simulink model "quadcoptermodel_liniarize"  (R2017b)
settings: Solver=FixedStepAuto  StartTime=0.0  StopTime=10.0  FixedStep=0.0025  RelTol=1e-3

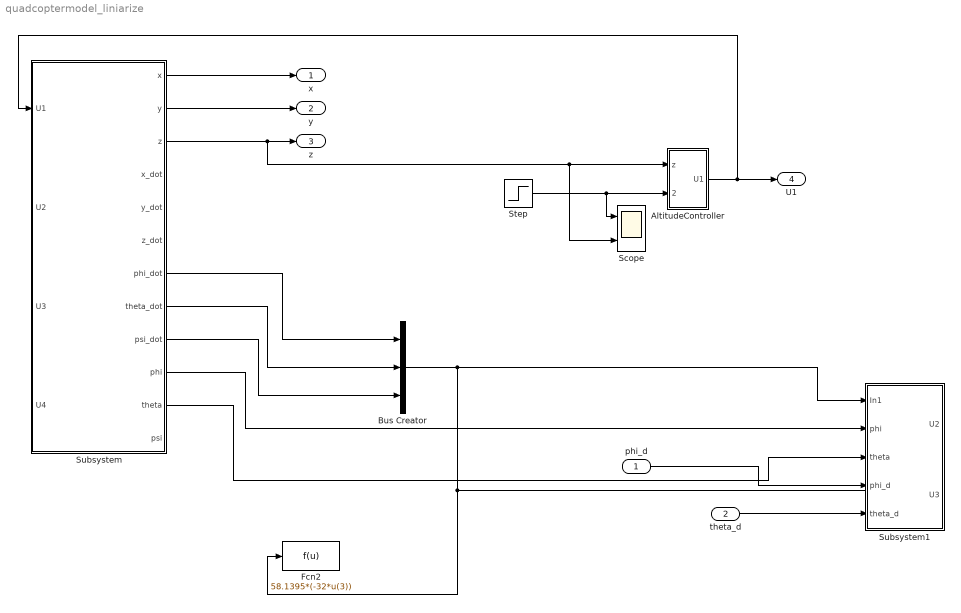
== system quadcoptermodel_liniarize ==
  phi_d : Inport
  theta_d : Inport  Port=2
  AltitudeController : Subsystem
  Bus Creator : BusCreator  Inputs=3
  Fcn2 : Fcn  Expr=58.1395*(-32*u(3))
  Scope : Scope  NumInputPorts=2
  Step : Step  SampleTime=0
  Subsystem : Subsystem
  Subsystem1 : Subsystem
  x : Outport
  y : Outport  Port=2
  z : Outport  Port=3
  U1 : Outport  Port=4
  wires:
  Subsystem/1(x) -> x/1
  Subsystem/2(y) -> y/1
  Subsystem/3(z) -> Scope/2, AltitudeController/1(z), z/1
  AltitudeController/1(U1) -> Subsystem/1(U1), U1/1
  Step/1 -> Scope/1, AltitudeController/2(z_d)
  Subsystem/7(phi_dot) -> Bus Creator/1
  Subsystem/8(theta_dot) -> Bus Creator/2
  Subsystem/9(psi_dot) -> Bus Creator/3
  Bus Creator/1 -> Subsystem1/1(In1), Fcn2/1
  Subsystem/10(phi) -> Subsystem1/2(phi)
  Subsystem/11(theta) -> Subsystem1/3(theta)
  phi_d/1 -> Subsystem1/4(phi_d)
  theta_d/1 -> Subsystem1/5(theta_d)

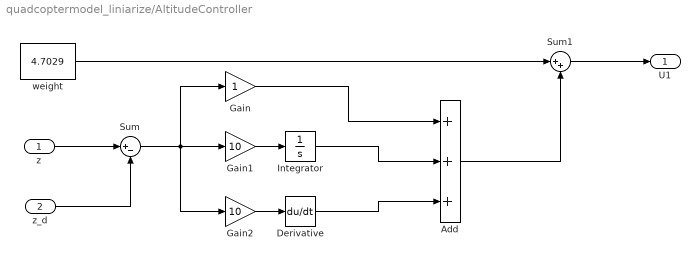
== system quadcoptermodel_liniarize/AltitudeController ==
  z : Inport
  z_d : Inport  Port=2
  Add : Sum  Inputs=+++
  Derivative : Derivative
  Gain : Gain
  Gain1 : Gain  Gain=10
  Gain2 : Gain  Gain=10
  Integrator : Integrator
  Sum : Sum  Inputs=|+-
  Sum1 : Sum  Inputs=|++
  weight : Constant  Value=4.7029
  U1 : Outport
  wires:
  Gain1/1 -> Integrator/1
  Sum/1 -> Gain/1, Gain1/1, Gain2/1
  weight/1 -> Sum1/1
  z_d/1 -> Sum/2
  Integrator/1 -> Add/2
  Add/1 -> Sum1/2
  Gain/1 -> Add/1
  Gain2/1 -> Derivative/1
  z/1 -> Sum/1
  Sum1/1 -> U1/1
  Derivative/1 -> Add/3

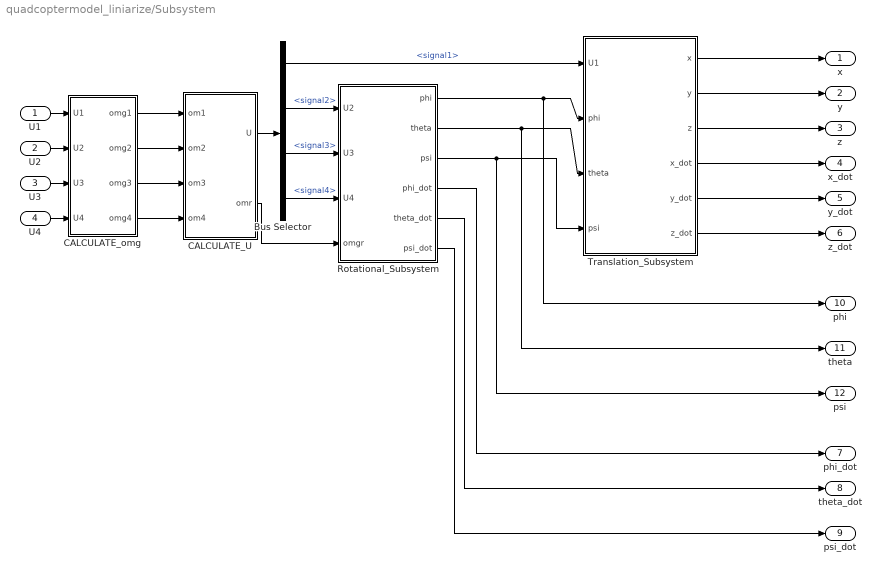
== system quadcoptermodel_liniarize/Subsystem ==
  U1 : Inport
  U2 : Inport  Port=2
  U3 : Inport  Port=3
  U4 : Inport  Port=4
  Bus Selector : BusSelector  OutputSignals=signal1,signal2,signal3,signal4
  CALCULATE_U : Subsystem
  CALCULATE_omg : Subsystem
  Rotational_Subsystem : Subsystem
  Translation_Subsystem : Subsystem
  x : Outport
  y : Outport  Port=2
  z : Outport  Port=3
  x_dot : Outport  Port=4
  y_dot : Outport  Port=5
  z_dot : Outport  Port=6
  phi_dot : Outport  Port=7
  theta_dot : Outport  Port=8
  psi_dot : Outport  Port=9
  phi : Outport  Port=10
  theta : Outport  Port=11
  psi : Outport  Port=12
  wires:
  CALCULATE_omg/1(omg1) -> CALCULATE_U/1(om1)
  CALCULATE_omg/4(omg4) -> CALCULATE_U/4(om4)
  CALCULATE_omg/2(omg2) -> CALCULATE_U/2(om2)
  CALCULATE_U/1(U) -> Bus Selector/1
  CALCULATE_omg/3(omg3) -> CALCULATE_U/3(om3)
  Rotational_Subsystem/1(phi) -> phi/1, Translation_Subsystem/2(phi)
  Rotational_Subsystem/2(theta) -> theta/1, Translation_Subsystem/3(theta)
  Rotational_Subsystem/3(psi) -> psi/1, Translation_Subsystem/4(psi)
  Translation_Subsystem/1(x) -> x/1
  Bus Selector/1 -> Translation_Subsystem/1(U1)  "<signal1>"
  Translation_Subsystem/2(y) -> y/1
  Translation_Subsystem/3(z) -> z/1
  Bus Selector/3 -> Rotational_Subsystem/2(U3)  "<signal3>"
  Bus Selector/4 -> Rotational_Subsystem/3(U4)  "<signal4>"
  CALCULATE_U/2(omr) -> Rotational_Subsystem/4(omgr)
  Bus Selector/2 -> Rotational_Subsystem/1(U2)  "<signal2>"
  Translation_Subsystem/6(z_dot) -> z_dot/1
  Translation_Subsystem/4(x_dot) -> x_dot/1
  U3/1 -> CALCULATE_omg/3(U3)
  Rotational_Subsystem/5(theta_dot) -> theta_dot/1
  U4/1 -> CALCULATE_omg/4(U4)
  U2/1 -> CALCULATE_omg/2(U2)
  U1/1 -> CALCULATE_omg/1(U1)
  Translation_Subsystem/5(y_dot) -> y_dot/1
  Rotational_Subsystem/6(psi_dot) -> psi_dot/1
  Rotational_Subsystem/4(phi_dot) -> phi_dot/1

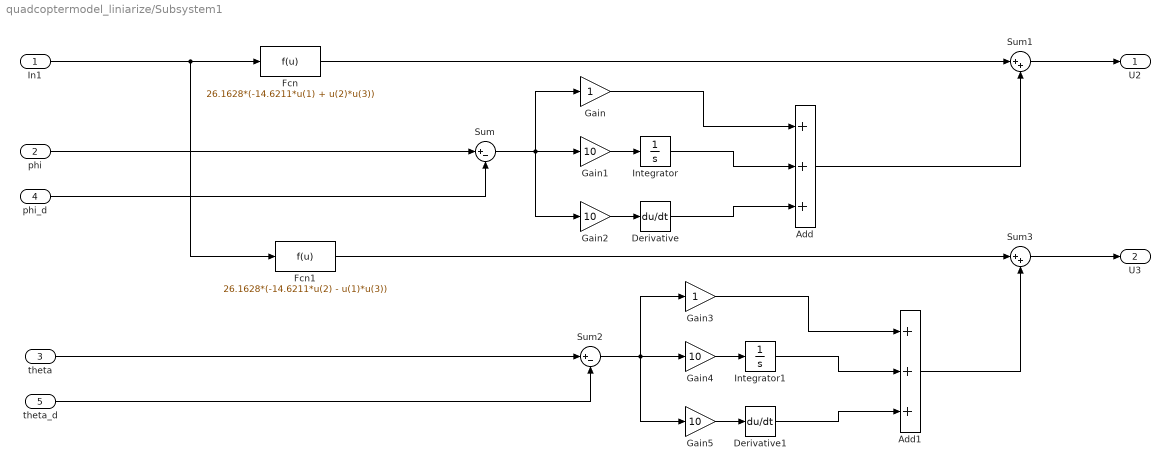
== system quadcoptermodel_liniarize/Subsystem1 ==
  In1 : Inport
  phi : Inport  Port=2
  theta : Inport  Port=3
  phi_d : Inport  Port=4
  theta_d : Inport  Port=5
  Add : Sum  Inputs=+++
  Add1 : Sum  Inputs=+++
  Derivative : Derivative
  Derivative1 : Derivative
  Fcn : Fcn  Expr=26.1628*(-14.6211*u(1) + u(2)*u(3))
  Fcn1 : Fcn  Expr=26.1628*(-14.6211*u(2) - u(1)*u(3))
  Gain : Gain
  Gain{1..2,4..5} (4 alike) : Gain  Gain=10
  Gain3 : Gain
  Integrator : Integrator
  Integrator1 : Integrator
  Sum : Sum  Inputs=|+-
  Sum1 : Sum  Inputs=|++
  Sum2 : Sum  Inputs=|+-
  Sum3 : Sum  Inputs=|++
  U2 : Outport
  U3 : Outport  Port=2
  wires:
  In1/1 -> Fcn1/1, Fcn/1
  theta_d/1 -> Sum2/2
  Integrator1/1 -> Add1/2
  Fcn1/1 -> Sum3/1
  Derivative1/1 -> Add1/3
  theta/1 -> Sum2/1
  Gain4/1 -> Integrator1/1
  Add1/1 -> Sum3/2
  Gain5/1 -> Derivative1/1
  Sum2/1 -> Gain3/1, Gain4/1, Gain5/1
  Sum3/1 -> U3/1
  Gain3/1 -> Add1/1
  Add/1 -> Sum1/2
  Integrator/1 -> Add/2
  phi_d/1 -> Sum/2
  Derivative/1 -> Add/3
  Gain/1 -> Add/1
  Gain2/1 -> Derivative/1
  Gain1/1 -> Integrator/1
  Sum/1 -> Gain/1, Gain1/1, Gain2/1
  Sum1/1 -> U2/1
  phi/1 -> Sum/1
  Fcn/1 -> Sum1/1

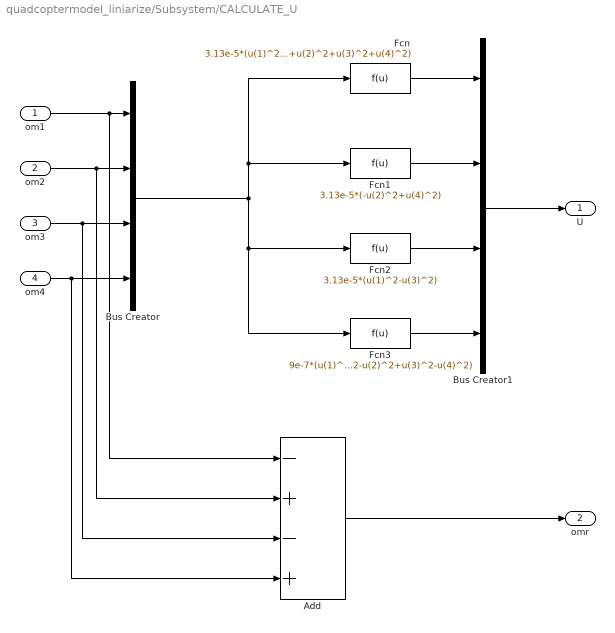
== system quadcoptermodel_liniarize/Subsystem/CALCULATE_U ==
  om1 : Inport
  om2 : Inport  Port=2
  om3 : Inport  Port=3
  om4 : Inport  Port=4
  Add : Sum  Inputs=-+-+
  Bus Creator : BusCreator  Inputs=4
  Bus Creator1 : BusCreator  Inputs=4
  Fcn : Fcn  Expr=3.13e-5*(u(1)^2+u(2)^2+u(3)^2+u(4)^2)
  Fcn1 : Fcn  Expr=3.13e-5*(-u(2)^2+u(4)^2)
  Fcn2 : Fcn  Expr=3.13e-5*(u(1)^2-u(3)^2)
  Fcn3 : Fcn  Expr=9e-7*(u(1)^2-u(2)^2+u(3)^2-u(4)^2)
  U : Outport
  omr : Outport  Port=2
  wires:
  Bus Creator1/1 -> U/1
  om3/1 -> Add/3, Bus Creator/3
  om1/1 -> Add/1, Bus Creator/1
  Bus Creator/1 -> Fcn3/1, Fcn2/1, Fcn1/1, Fcn/1
  Fcn1/1 -> Bus Creator1/2
  om4/1 -> Add/4, Bus Creator/4
  Fcn/1 -> Bus Creator1/1
  Fcn2/1 -> Bus Creator1/3
  om2/1 -> Add/2, Bus Creator/2
  Fcn3/1 -> Bus Creator1/4
  Add/1 -> omr/1

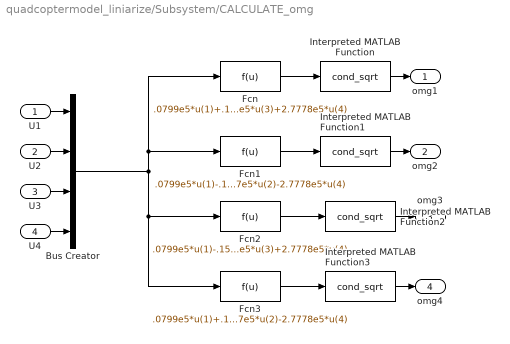
== system quadcoptermodel_liniarize/Subsystem/CALCULATE_omg ==
  U1 : Inport
  U2 : Inport  Port=2
  U3 : Inport  Port=3
  U4 : Inport  Port=4
  Bus Creator : BusCreator  Inputs=4
  Fcn : Fcn  Expr=.0799e5*u(1)+.1597e5*u(3)+2.7778e5*u(4)
  Fcn1 : Fcn  Expr=.0799e5*u(1)-.1597e5*u(2)-2.7778e5*u(4)
  Fcn2 : Fcn  Expr=.0799e5*u(1)-.1597e5*u(3)+2.7778e5*u(4)
  Fcn3 : Fcn  Expr=.0799e5*u(1)+.1597e5*u(2)-2.7778e5*u(4)
  Interpreted MATLAB Function{,1..3} (4 alike) : MATLABFcn  MATLABFcn=cond_sqrt
  omg1 : Outport
  omg2 : Outport  Port=2
  omg3 : Outport  Port=3
  omg4 : Outport  Port=4
  wires:
  Fcn/1 -> Interpreted MATLAB Function/1
  Fcn3/1 -> Interpreted MATLAB Function3/1
  U3/1 -> Bus Creator/3
  U4/1 -> Bus Creator/4
  Interpreted MATLAB Function/1 -> omg1/1
  Interpreted MATLAB Function3/1 -> omg4/1
  Interpreted MATLAB Function2/1 -> omg3/1
  Interpreted MATLAB Function1/1 -> omg2/1
  U1/1 -> Bus Creator/1
  U2/1 -> Bus Creator/2
  Fcn1/1 -> Interpreted MATLAB Function1/1
  Fcn2/1 -> Interpreted MATLAB Function2/1
  Bus Creator/1 -> Fcn2/1, Fcn3/1, Fcn1/1, Fcn/1

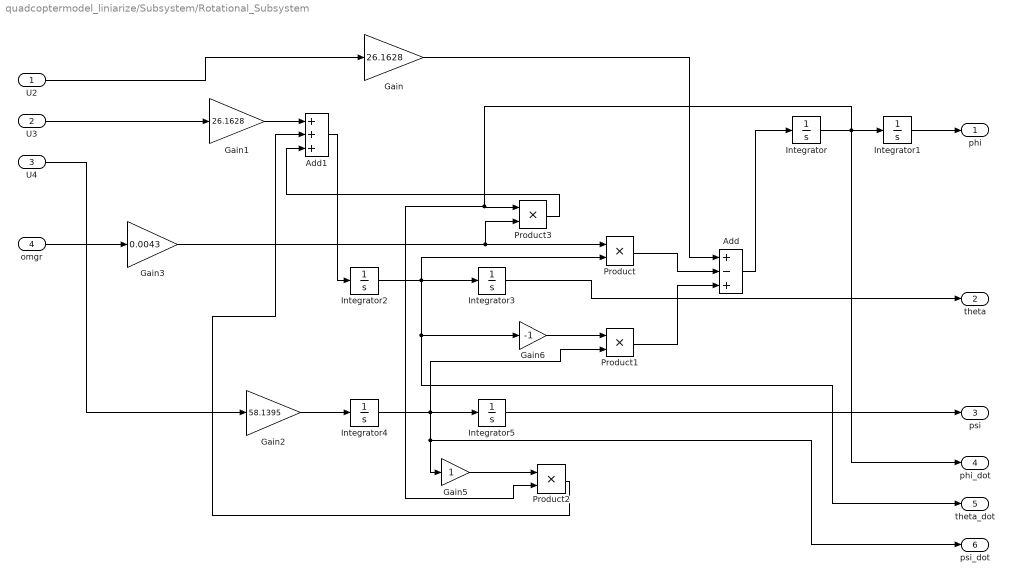
== system quadcoptermodel_liniarize/Subsystem/Rotational_Subsystem ==
  U2 : Inport
  U3 : Inport  Port=2
  U4 : Inport  Port=3
  omgr : Inport  Port=4
  Add : Sum  Inputs=+-+
  Add1 : Sum  Inputs=+++
  Gain : Gain  Gain=26.1628
  Gain1 : Gain  Gain=26.1628
  Gain2 : Gain  Gain=58.1395
  Gain3 : Gain  Gain=0.0043
  Gain5 : Gain
  Gain6 : Gain  Gain=-1
  Integrator{,1..5} (6 alike) : Integrator
  Product{,1..3} (4 alike) : Product
  phi : Outport
  theta : Outport  Port=2
  psi : Outport  Port=3
  phi_dot : Outport  Port=4
  theta_dot : Outport  Port=5
  psi_dot : Outport  Port=6
  wires:
  Gain3/1 -> Product3/2, Product/1
  Integrator2/1 -> theta_dot/1, Gain6/1, Product/2, Integrator3/1
  Product1/1 -> Add/3
  Integrator1/1 -> phi/1
  Integrator4/1 -> psi_dot/1, Gain5/1, Product1/2, Integrator5/1
  U4/1 -> Gain2/1
  Integrator5/1 -> psi/1
  Integrator/1 -> phi_dot/1, Product2/2, Product3/1, Integrator1/1
  U2/1 -> Gain/1
  Gain2/1 -> Integrator4/1
  Gain5/1 -> Product2/1
  Add/1 -> Integrator/1
  U3/1 -> Gain1/1
  Gain/1 -> Add/1
  Gain6/1 -> Product1/1
  Product/1 -> Add/2
  Integrator3/1 -> theta/1
  Product2/1 -> Add1/2
  Gain1/1 -> Add1/1
  Product3/1 -> Add1/3
  Add1/1 -> Integrator2/1
  omgr/1 -> Gain3/1

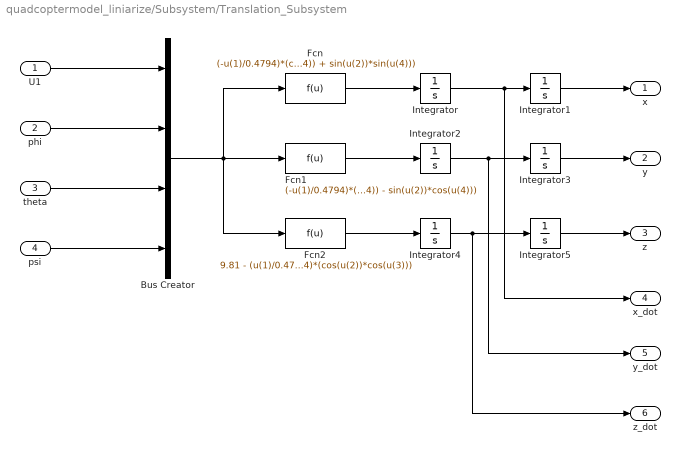
== system quadcoptermodel_liniarize/Subsystem/Translation_Subsystem ==
  U1 : Inport
  phi : Inport  Port=2
  theta : Inport  Port=3
  psi : Inport  Port=4
  Bus Creator : BusCreator  Inputs=4
  Fcn : Fcn  Expr=(-u(1)/0.4794)*(cos(u(2))*sin(u(3))*cos(u(4)) + sin(u(2))*sin(u(4)))
  Fcn1 : Fcn  Expr=(-u(1)/0.4794)*(cos(u(2))*sin(u(3))*sin(u(4)) - sin(u(2))*cos(u(4)))
  Fcn2 : Fcn  Expr=9.81 - (u(1)/0.4794)*(cos(u(2))*cos(u(3)))
  Integrator{,1..5} (6 alike) : Integrator
  x : Outport
  y : Outport  Port=2
  z : Outport  Port=3
  x_dot : Outport  Port=4
  y_dot : Outport  Port=5
  z_dot : Outport  Port=6
  wires:
  U1/1 -> Bus Creator/1
  Integrator5/1 -> z/1
  Integrator1/1 -> x/1
  Bus Creator/1 -> Fcn2/1, Fcn1/1, Fcn/1
  psi/1 -> Bus Creator/4
  phi/1 -> Bus Creator/2
  theta/1 -> Bus Creator/3
  Fcn/1 -> Integrator/1
  Fcn1/1 -> Integrator2/1
  Integrator2/1 -> y_dot/1, Integrator3/1
  Integrator/1 -> x_dot/1, Integrator1/1
  Fcn2/1 -> Integrator4/1
  Integrator4/1 -> z_dot/1, Integrator5/1
  Integrator3/1 -> y/1
